simulink model "Emmanuel_Mati_Simulink_Project_Unit_Ramp_Input"  (R2020a)
settings: Solver=VariableStepAuto  StartTime=0.0  StopTime=10  RelTol=1e-3
libraries: simulink x3
settings Model: Creator=mati1  LastModifiedBy=mati1

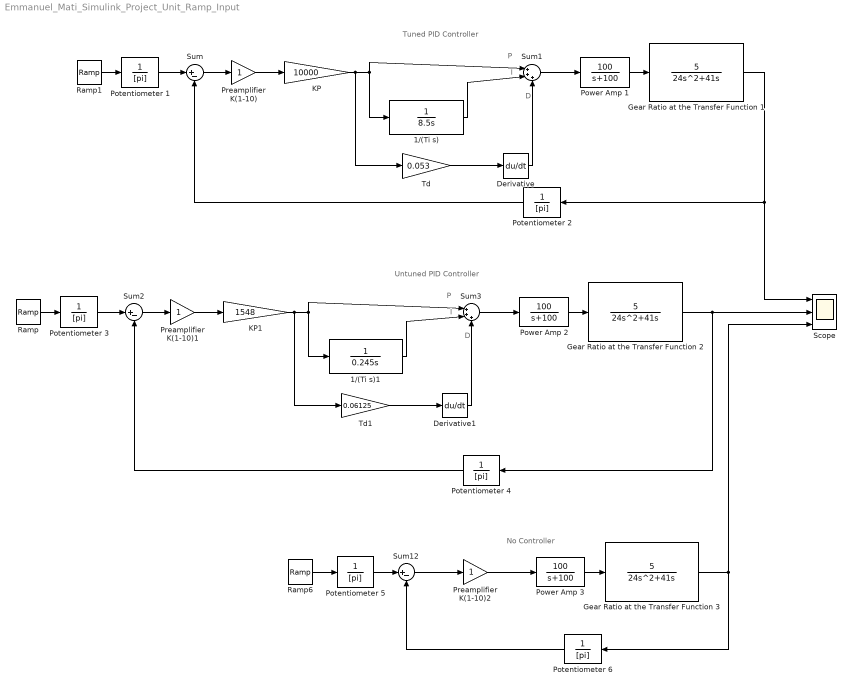
== system Emmanuel_Mati_Simulink_Project_Unit_Ramp_Input ==
  note: No Controller
  note: Untuned PID Controller
  note: Tuned PID Controller
  note: I
  note: P
  note: D
  note: I
  note: P
  note: D
  1/(Ti s) : TransferFcn  Denominator=[8.5 0]
  1/(Ti s)1 : TransferFcn  Denominator=[0.245 0]
  Derivative : Derivative
  Derivative1 : Derivative
  Gear Ratio at the Transfer Function 1 : TransferFcn  Numerator=[5]  Denominator=[24 41 0]
  Gear Ratio at the Transfer Function 2 : TransferFcn  Numerator=[5]  Denominator=[24 41 0]
  Gear Ratio at the Transfer Function 3 : TransferFcn  Numerator=[5]  Denominator=[24 41 0]
  KP : Gain  Gain=10000
  KP1 : Gain  Gain=1548
  Potentiometer {1..6} (6 alike) : TransferFcn  Denominator=[pi]
  Power Amp 1 : TransferFcn  Numerator=[100]  Denominator=[1 100]
  Power Amp 2 : TransferFcn  Numerator=[100]  Denominator=[1 100]
  Power Amp 3 : TransferFcn  Numerator=[100]  Denominator=[1 100]
  Preamplifier K(1-10) : Gain
  Preamplifier K(1-10)1 : Gain
  Preamplifier K(1-10)2 : Gain
  Ramp : simulink/Sources/Ramp  slope=1  start=0  InitialOutput=0
  Ramp1 : simulink/Sources/Ramp  slope=1  start=0  InitialOutput=0
  Ramp6 : simulink/Sources/Ramp  slope=1  start=0  InitialOutput=0
  Scope : Scope  NumInputPorts=3
  Sum : Sum  Inputs=|+-
  Sum1 : Sum  Inputs=|+++
  Sum12 : Sum  Inputs=|+-
  Sum2 : Sum  Inputs=|+-
  Sum3 : Sum  Inputs=|+++
  Td : Gain  Gain=0.053
  Td1 : Gain  Gain=0.06125
  wires:
  KP/1 -> Td/1, 1/(Ti s)/1, Sum1/1
  Sum1/1 -> Power Amp 1/1
  1/(Ti s)/1 -> Sum1/2
  Td/1 -> Derivative/1
  Preamplifier K(1-10)/1 -> KP/1
  Derivative/1 -> Sum1/3
  Sum/1 -> Preamplifier K(1-10)/1
  Gear Ratio at the Transfer Function 1/1 -> Potentiometer 2/1, Scope/1
  Ramp1/1 -> Potentiometer 1/1
  Power Amp 1/1 -> Gear Ratio at the Transfer Function 1/1
  Potentiometer 1/1 -> Sum/1
  Potentiometer 2/1 -> Sum/2
  Sum3/1 -> Power Amp 2/1
  Potentiometer 4/1 -> Sum2/2
  Potentiometer 3/1 -> Sum2/1
  Power Amp 2/1 -> Gear Ratio at the Transfer Function 2/1
  Td1/1 -> Derivative1/1
  Ramp/1 -> Potentiometer 3/1
  Sum2/1 -> Preamplifier K(1-10)1/1
  Preamplifier K(1-10)1/1 -> KP1/1
  Gear Ratio at the Transfer Function 2/1 -> Scope/2, Potentiometer 4/1
  KP1/1 -> Td1/1, 1/(Ti s)1/1, Sum3/1
  Derivative1/1 -> Sum3/3
  1/(Ti s)1/1 -> Sum3/2
  Ramp6/1 -> Potentiometer 5/1
  Preamplifier K(1-10)2/1 -> Power Amp 3/1
  Sum12/1 -> Preamplifier K(1-10)2/1
  Gear Ratio at the Transfer Function 3/1 -> Scope/3, Potentiometer 6/1
  Power Amp 3/1 -> Gear Ratio at the Transfer Function 3/1
  Potentiometer 5/1 -> Sum12/1
  Potentiometer 6/1 -> Sum12/2
